simulink model "omnibundle"  (R2018b)
settings: Solver=ode2  StartTime=0.0  StopTime=40  FixedStep=0.01  RelTol=1e-3
values from neighbouring files (symbols this model uses):
  dq0 = [0.1 0 0]'    [main.m]    (also in main_noL.m)
  q0 = [pi/6; -pi/3; 0; -pi/3; -pi/6; pi/2; pi/2]    [Lab1__KUKA__IIWA14.m]    (also in main.m = [0 0 0]'; main_noL.m = [0 0 0]')
settings Model: Creator=Renata  LastModifiedBy=Renata

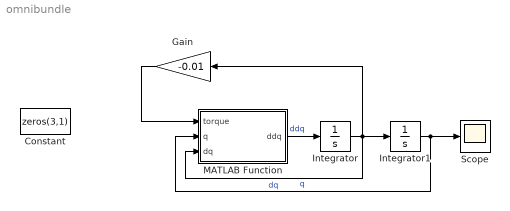
== system omnibundle ==
  Constant : Constant  Value=zeros(3,1)
  Gain : Gain  Gain=-0.01
  Integrator : Integrator  InitialCondition=dq0
  Integrator1 : Integrator  InitialCondition=q0
  MATLAB Function : MATLAB Function  TreatAsAtomicUnit=on
  Scope : Scope
  wires:
  MATLAB Function/1(ddq) -> Integrator/1  "ddq"
  Integrator1/1 -> MATLAB Function/2(q), Scope/1  "q"
  Gain/1 -> MATLAB Function/1(torque)
  Integrator/1 -> Gain/1, MATLAB Function/3(dq), Integrator1/1  "dq"

== matlab function omnibundle/MATLAB Function ==
  data: torque input; q input; dq input; ddq output
function ddq = fcn(torque,q,dq)
    
    ddq = dyn_omni_bundle_fun(9.8, q, dq, torque);
